simulink model "Laengsdynamik"  (R2020b)
settings: Solver=FixedStepAuto  StartTime=0.0  StopTime=60  RelTol=1e-3
settings Model: Creator=62958  LastModifiedBy=62958
settings HardwareCC: ProdHWDeviceType=AMD->x86-64 (Windows64)

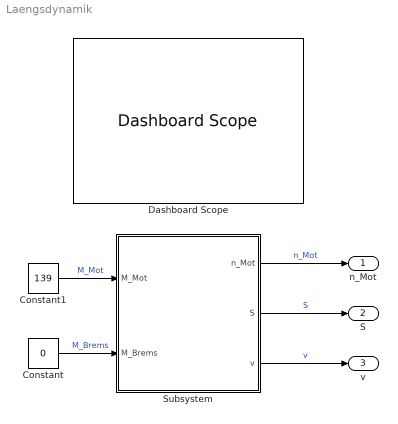
== system Laengsdynamik ==
  Constant : Constant  Value=0
  Constant1 : Constant  Value=139
  Dashboard Scope : DashboardScope  LegendPosition=Right
  Subsystem : Subsystem
  n_Mot : Outport
  S : Outport  Port=2
  v : Outport  Port=3
  wires:
  Constant1/1 -> Subsystem/1(M_Mot)  "M_Mot"
  Constant/1 -> Subsystem/2(M_Brems)  "M_Brems"
  Subsystem/1(n_Mot) -> n_Mot/1  "n_Mot"
  Subsystem/2(S) -> S/1  "S"
  Subsystem/3(v) -> v/1  "v"

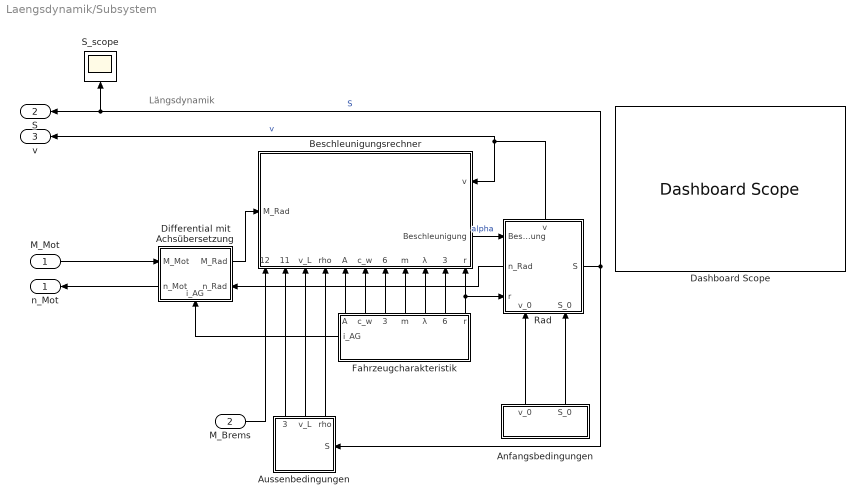
== system Laengsdynamik/Subsystem ==
  note: Längsdynamik
  M_Mot : Inport
  M_Brems : Inport  Port=2
  Anfangsbedingungen : Subsystem
  Aussenbedingungen : Subsystem
      settings: PortSchema="{\"entries\":[{\"content\":{\"sides\":[{\"content\":{\"connectorIds\":[\"In1\"]},\"type\":\"ConnectorPlacement.EquallySpacedRectSide\",\"uuid\":\"b733fa8f-5d00-494c-b34f-88b15d5a1e12\"},{\"content\":{\"connectorIds\":[],\"side\":\"RIGHT\"},\"type\":\"ConnectorPlacement.EquallySpacedRectSide\",\"uuid\":\"0860ef04-b928-4d53-b793-a96484e4cbe0\"},{\"content\":{\"connectorIds\":[\"Out1\",\"Out2\",\"Out3\"],\"side\":\"TOP\"},\"type\":\"ConnectorPlacement.EquallySpacedRectSide\",\"uuid\":\"090c1db3-6356-4eaa-9d0b-055902e2f27b\"},{\"content\":{\"connectorIds\":[],\"side\":\"BOTTOM\"},\"type\":\"ConnectorPlacement.EquallySpacedRectSide\",\"uuid\":\"59190b0a-2250-4f57-8c29-4644eef2c409\"},{\"content\":{\"connectorIds\":[],\"side\":\"HIDDEN\"},\"type\":\"ConnectorPlacement.EquallySpacedRectSide\",\"uuid\":\"ec20f46d-06e3-4d0a-9c7e-927ffb9f63c9\"}]},\"type\":\"ConnectorPlacement.EquallySpacedConnector\",\"uuid\":\"5c9482c8-38cc-4f92-88a5-86b3dbc9bf94\"}],\"packageUris\":[\"http://schema.mathworks.com/mf0/Connector/R2020b\"],\"version\":\"1.0\"}"
  Beschleunigungsrechner : Subsystem
      settings: PortSchema="{\"entries\":[{\"content\":{\"sides\":[{\"content\":{\"connectorIds\":[\"In1\",\"Out1\"]},\"type\":\"ConnectorPlacement.EquallySpacedRectSide\",\"uuid\":\"b733fa8f-5d00-494c-b34f-88b15d5a1e12\"},{\"content\":{\"connectorIds\":[\"In13\"],\"side\":\"RIGHT\"},\"type\":\"ConnectorPlacement.EquallySpacedRectSide\",\"uuid\":\"0860ef04-b928-4d53-b793-a96484e4cbe0\"},{\"content\":{\"connectorIds\":[],\"side\":\"TOP\"},\"type\":\"ConnectorPlacement.EquallySpacedRectSide\",\"uuid\":\"090c1db3-6356-4eaa-9d0b-055902e2f27b\"},{\"content\":{\"connectorIds\":[\"In2\",\"In3\",\"In4\",\"In5\",\"In6\",\"In7\",\"In8\",\"In9\",\"In10\",\"In11\",\"In12\"],\"side\":\"BOTTOM\"},\"type\":\"ConnectorPlacement.EquallySpacedRectSide\",\"uuid\":\"59190b0a-2250-4f57-8c29-4644eef2c409\"},{\"content\":{\"connectorIds\":[],\"side\":\"HIDDEN\"},\"type\":\"ConnectorPlacement.EquallySpacedRectSide\",\"uuid\":\"ec20f46d-06e3-4d0a-9c7e-927ffb9f63c9\"}]},\"type\":\"ConnectorPlacement.EquallySpacedConnector\",\"uuid\":\"5c9482c8-38cc-4f92-88a5-86b3dbc9bf94\"}],\"packageUris\":[\"http://schema.mathworks.com/mf0/Connector/R2020b\"],\"version\":\"1.0\"}"
  Dashboard Scope : DashboardScope
  Differential mit Achsübersetzung : Subsystem
      settings: PortSchema="{\"entries\":[{\"content\":{\"sides\":[{\"content\":{\"connectorIds\":[\"In1\",\"Out2\"]},\"type\":\"ConnectorPlacement.EquallySpacedRectSide\",\"uuid\":\"b733fa8f-5d00-494c-b34f-88b15d5a1e12\"},{\"content\":{\"connectorIds\":[\"Out1\",\"In3\"],\"side\":\"RIGHT\"},\"type\":\"ConnectorPlacement.EquallySpacedRectSide\",\"uuid\":\"0860ef04-b928-4d53-b793-a96484e4cbe0\"},{\"content\":{\"connectorIds\":[],\"side\":\"TOP\"},\"type\":\"ConnectorPlacement.EquallySpacedRectSide\",\"uuid\":\"090c1db3-6356-4eaa-9d0b-055902e2f27b\"},{\"content\":{\"connectorIds\":[\"In2\"],\"side\":\"BOTTOM\"},\"type\":\"ConnectorPlacement.EquallySpacedRectSide\",\"uuid\":\"88222426-d39d-4ff1-9ccf-26b03ee0e8eb\"},{\"content\":{\"connectorIds\":[],\"side\":\"HIDDEN\"},\"type\":\"ConnectorPlacement.EquallySpacedRectSide\",\"uuid\":\"ec20f46d-06e3-4d0a-9c7e-927ffb9f63c9\"}]},\"type\":\"ConnectorPlacement.EquallySpacedConnector\",\"uuid\":\"5c9482c8-38cc-4f92-88a5-86b3dbc9bf94\"}],\"packageUris\":[\"http://schema.mathworks.com/mf0/Connector/R2020b\"],\"version\":\"1.0\"}"
  Fahrzeugcharakteristik : Subsystem
      settings: PortSchema="{\"entries\":[{\"content\":{\"sides\":[{\"content\":{\"connectorIds\":[\"Out8\"]},\"type\":\"ConnectorPlacement.EquallySpacedRectSide\",\"uuid\":\"425210de-c24d-4735-89d6-da620fee91ae\"},{\"content\":{\"connectorIds\":[],\"side\":\"RIGHT\"},\"type\":\"ConnectorPlacement.EquallySpacedRectSide\",\"uuid\":\"2aa95b8b-744b-4218-9974-9819eac83ec9\"},{\"content\":{\"connectorIds\":[\"Out1\",\"Out2\",\"Out3\",\"Out4\",\"Out5\",\"Out6\",\"Out7\"],\"side\":\"TOP\"},\"type\":\"ConnectorPlacement.EquallySpacedRectSide\",\"uuid\":\"44fb0172-403e-4023-85b6-026c89d7dec6\"},{\"content\":{\"connectorIds\":[],\"side\":\"HIDDEN\"},\"type\":\"ConnectorPlacement.EquallySpacedRectSide\",\"uuid\":\"03215e6b-5de7-4733-a8b0-f647922a7984\"}]},\"type\":\"ConnectorPlacement.EquallySpacedConnector\",\"uuid\":\"d1bd5eef-fe53-4c9e-be8a-2ad764aa59c2\"}],\"packageUris\":[\"http://schema.mathworks.com/mf0/Connector/R2020b\"],\"version\":\"1.0\"}"
  Rad : Subsystem
      settings: PortSchema="{\"entries\":[{\"content\":{\"sides\":[{\"content\":{\"connectorIds\":[\"In1\",\"Out3\",\"In2\"]},\"type\":\"ConnectorPlacement.EquallySpacedRectSide\",\"uuid\":\"c3417092-dc7c-4039-9e9c-c2a6b9640efa\"},{\"content\":{\"connectorIds\":[\"Out1\"],\"side\":\"RIGHT\"},\"type\":\"ConnectorPlacement.EquallySpacedRectSide\",\"uuid\":\"749acbb4-c656-4eff-a125-532591d5cf60\"},{\"content\":{\"connectorIds\":[\"Out2\"],\"side\":\"TOP\"},\"type\":\"ConnectorPlacement.EquallySpacedRectSide\",\"uuid\":\"92c07f50-a812-457a-9ad7-17c408d902db\"},{\"content\":{\"connectorIds\":[\"In3\",\"In4\"],\"side\":\"BOTTOM\"},\"type\":\"ConnectorPlacement.EquallySpacedRectSide\",\"uuid\":\"b98cd1e8-b633-4d79-aeaf-c664ca03f589\"},{\"content\":{\"connectorIds\":[],\"side\":\"HIDDEN\"},\"type\":\"ConnectorPlacement.EquallySpacedRectSide\",\"uuid\":\"4099a9b5-4655-4782-9301-3d866c99b02b\"}]},\"type\":\"ConnectorPlacement.EquallySpacedConnector\",\"uuid\":\"1fc2dbdd-5020-4d82-be08-5c03d0ed68f0\"}],\"packageUris\":[\"http://schema.mathworks.com/mf0/Connector/R2020b\"],\"version\":\"1.0\"}"
  S_scope : Scope
  n_Mot : Outport
  S : Outport  Port=2
  v : Outport  Port=3
  wires:
  Fahrzeugcharakteristik/7(r) -> Beschleunigungsrechner/2(r), Rad/2(r)
  Fahrzeugcharakteristik/4(m) -> Beschleunigungsrechner/5(m)
  M_Mot/1 -> Differential mit Achsübersetzung/1(M_Mot)
  Aussenbedingungen/2(v_L) -> Beschleunigungsrechner/10(v_L)
  Rad/2(v) -> v/1, Beschleunigungsrechner/1(v)  "v"
  Rad/1(S) -> Aussenbedingungen/1(S), S/1, S_scope/1  "S"
  Beschleunigungsrechner/1(Beschleunigung) -> Rad/1(Beschleunigung)  "alpha"
  M_Brems/1 -> Beschleunigungsrechner/12(M_Brems)
  Differential mit Achsübersetzung/2(n_Mot) -> n_Mot/1
  Aussenbedingungen/3(gamma) -> Beschleunigungsrechner/11(gamma)
  Rad/3(n_Rad) -> Differential mit Achsübersetzung/3(n_Rad)
  Fahrzeugcharakteristik/8(i_AG) -> Differential mit Achsübersetzung/2(i_AG)
  Anfangsbedingungen/1(v_0) -> Rad/3(v_0)
  Aussenbedingungen/1(rho) -> Beschleunigungsrechner/9(rho)
  Differential mit Achsübersetzung/1(M_Rad) -> Beschleunigungsrechner/13(M_Rad)
  Fahrzeugcharakteristik/5(λ) -> Beschleunigungsrechner/4(λ)
  Fahrzeugcharakteristik/2(c_w) -> Beschleunigungsrechner/7(c_w)
  Fahrzeugcharakteristik/1(A) -> Beschleunigungsrechner/8(A)
  Anfangsbedingungen/2(S_0) -> Rad/4(S_0)
  Fahrzeugcharakteristik/6(F_Reib) -> Beschleunigungsrechner/3(F_Reib)
  Fahrzeugcharakteristik/3(f_Roll) -> Beschleunigungsrechner/6(f_Roll)

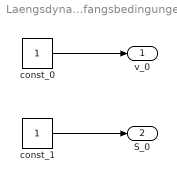
== system Laengsdynamik/Subsystem/Anfangsbedingungen ==
  const_0 : Constant
  const_1 : Constant
  v_0 : Outport
  S_0 : Outport  Port=2
  wires:
  const_1/1 -> S_0/1
  const_0/1 -> v_0/1

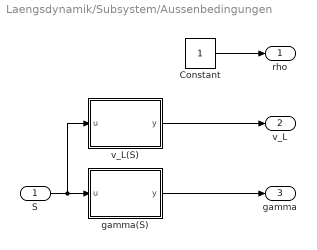
== system Laengsdynamik/Subsystem/Aussenbedingungen ==
  S : Inport
  Constant : Constant
  gamma(S) : MATLAB Function  TreatAsAtomicUnit=on
  v_L(S) : MATLAB Function  TreatAsAtomicUnit=on
  rho : Outport
  v_L : Outport  Port=2
  gamma : Outport  Port=3
  wires:
  Constant/1 -> rho/1
  gamma(S)/1(y) -> gamma/1
  v_L(S)/1(y) -> v_L/1
  S/1 -> v_L(S)/1(u), gamma(S)/1(u)

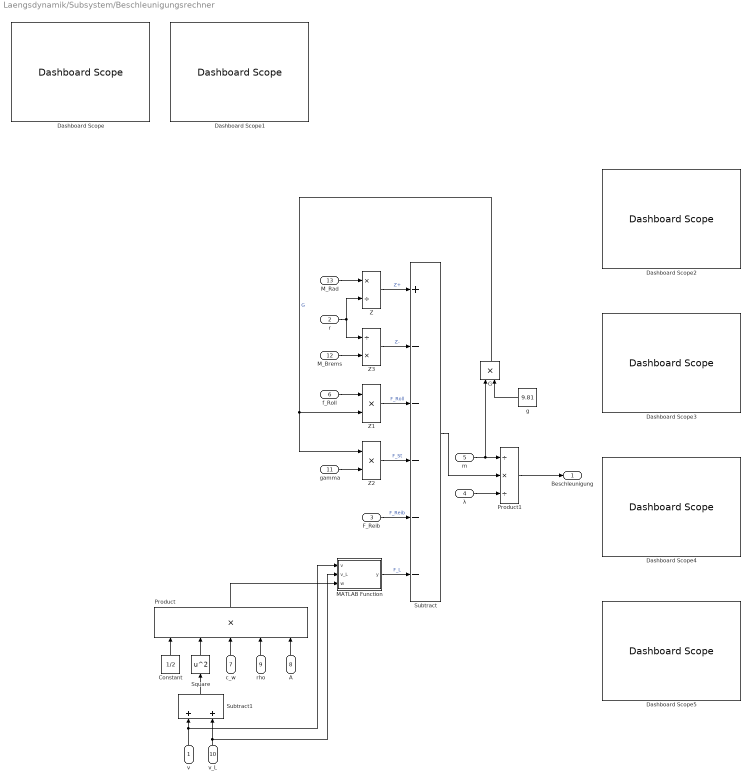
== system Laengsdynamik/Subsystem/Beschleunigungsrechner ==
  v : Inport
  r : Inport  Port=2
  F_Reib : Inport  Port=3
  λ : Inport  Port=4
  m : Inport  Port=5
  f_Roll : Inport  Port=6
  c_w : Inport  Port=7
  A : Inport  Port=8
  rho : Inport  Port=9
  v_L : Inport  Port=10
  gamma : Inport  Port=11
  M_Brems : Inport  Port=12
  M_Rad : Inport  Port=13
  Constant : Constant  Value=1/2
  Dashboard Scope : DashboardScope  Ymin=0  Ymax=150
  Dashboard Scope{1..5} (5 alike) : DashboardScope
  G : Product
  MATLAB Function : MATLAB Function  TreatAsAtomicUnit=on
  Product : Product  Inputs=5
  Product1 : Product  Inputs=/*/
  Square : Math  Operator=square  SaturateOnIntegerOverflow=on
  Subtract : Sum  Inputs=+-----
  Subtract1 : Sum
  Z : Product  Inputs=*/
  Z1 : Product  Inputs=**
  Z2 : Product  Inputs=**
  Z3 : Product  Inputs=/*
  g : Constant  Value=9.81
  Beschleunigung : Outport
  wires:
  M_Rad/1 -> Z/1
  r/1 -> Z3/1, Z/2
  Z/1 -> Subtract/1  "Z+"
  Product1/1 -> Beschleunigung/1
  Subtract/1 -> Product1/2
  m/1 -> G/1, Product1/1
  λ/1 -> Product1/3
  g/1 -> G/2
  G/1 -> Z2/1, Z1/2  "G"
  Z1/1 -> Subtract/3  "F_Roll"
  f_Roll/1 -> Z1/1
  gamma/1 -> Z2/2
  Z2/1 -> Subtract/4  "F_St"
  M_Brems/1 -> Z3/2
  Z3/1 -> Subtract/2  "Z-"
  v_L/1 -> Subtract1/2, MATLAB Function/2(v_L)
  v/1 -> MATLAB Function/1(v), Subtract1/1
  Subtract1/1 -> Square/1
  Constant/1 -> Product/1
  Square/1 -> Product/2
  c_w/1 -> Product/3
  rho/1 -> Product/4
  A/1 -> Product/5
  Product/1 -> MATLAB Function/3(w)
  F_Reib/1 -> Subtract/5  "F_Reib"
  MATLAB Function/1(y) -> Subtract/6  "F_L"

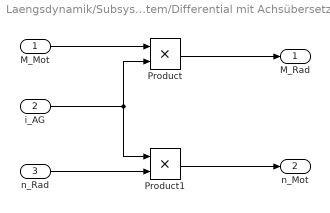
== system Laengsdynamik/Subsystem/Differential mit Achsübersetzung ==
  M_Mot : Inport
  i_AG : Inport  Port=2
  n_Rad : Inport  Port=3
  Product : Product
  Product1 : Product
  M_Rad : Outport
  n_Mot : Outport  Port=2
  wires:
  Product/1 -> M_Rad/1
  Product1/1 -> n_Mot/1
  M_Mot/1 -> Product/1
  i_AG/1 -> Product1/1, Product/2
  n_Rad/1 -> Product1/2

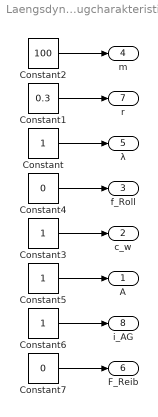
== system Laengsdynamik/Subsystem/Fahrzeugcharakteristik ==
  Constant{,3,5..6} (4 alike) : Constant
  Constant1 : Constant  Value=0.3
  Constant2 : Constant  Value=100
  Constant4 : Constant  Value=0
  Constant7 : Constant  Value=0
  A : Outport
  c_w : Outport  Port=2
  f_Roll : Outport  Port=3
  m : Outport  Port=4
  λ : Outport  Port=5
  F_Reib : Outport  Port=6
  r : Outport  Port=7
  i_AG : Outport  Port=8
  wires:
  Constant/1 -> λ/1
  Constant2/1 -> m/1
  Constant1/1 -> r/1
  Constant3/1 -> c_w/1
  Constant4/1 -> f_Roll/1
  Constant5/1 -> A/1
  Constant6/1 -> i_AG/1
  Constant7/1 -> F_Reib/1

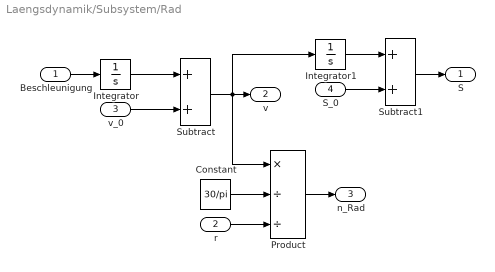
== system Laengsdynamik/Subsystem/Rad ==
  Beschleunigung : Inport
  r : Inport  Port=2
  v_0 : Inport  Port=3
  S_0 : Inport  Port=4
  Constant : Constant  Value=30/pi
  Integrator : Integrator
  Integrator1 : Integrator
  Product : Product  Inputs=*//
  Subtract : Sum
  Subtract1 : Sum
  S : Outport
  v : Outport  Port=2
  n_Rad : Outport  Port=3
  wires:
  Beschleunigung/1 -> Integrator/1
  Subtract/1 -> Product/1, Integrator1/1, v/1
  Integrator/1 -> Subtract/1
  v_0/1 -> Subtract/2
  S_0/1 -> Subtract1/2
  Integrator1/1 -> Subtract1/1
  Subtract1/1 -> S/1
  Constant/1 -> Product/2
  r/1 -> Product/3
  Product/1 -> n_Rad/1

== matlab function Laengsdynamik/Subsystem/Beschleunigungsrechner/MATLAB Function ==
  data: v input; v_L input; y output; w input
function y = fcn(v,v_L,w)
if v>v_L
    y=w;
elseif v<v_L
    y=-w;
else
    y=0;
end

== matlab function Laengsdynamik/Subsystem/Aussenbedingungen/v_L(S) ==
  data: u input; y output
function y = fcn(u)

y = 0.001*sin(u);

== matlab function Laengsdynamik/Subsystem/Aussenbedingungen/gamma(S) ==
  data: u input; y output
function y = fcn(u)

y = 0.001*sin(u);
